simulink model "test"  (R2015a)
settings: Solver=ode45  StartTime=0.0  StopTime=380000  RelTol=1e-3
InitFcn:
  | %% DSPBuilder Start
  | alt_dspbuilder_update_model(bdroot)
  | %% DSPBuilder End
libraries: allblocks_alteradspbuilder2 x2155
(part 1 of 24)
settings Model: Creator=ASUS  LastModifiedBy=ASUS

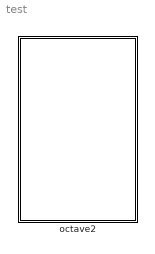
== system test ==
  octave2 : Subsystem

== system test/octave2 ==
  AltBus : allblocks_alteradspbuilder2/AltBus  BusType=Unsigned Integer  bwl=128  bwr=0  saturate=off  floatingPointInput=on  floatingPointOutput=on  logOutputs=off  logFile=C:\Users\ASUS\Desktop\sift_fpga_final\Octave_2\tb_test\test_octave2_AltBus.fixedpointlog
  AltBus1 : allblocks_alteradspbuilder2/AltBus  BusType=Unsigned Integer  bwl=1173  bwr=0  saturate=off  floatingPointInput=on  floatingPointOutput=on  logOutputs=off  logFile=C:\Users\ASUS\Desktop\sift_fpga_final\Octave_2\tb_test\test_octave2_AltBus1.fixedpointlog
  Bus_Concatenation : Subsystem
  Delay : allblocks_alteradspbuilder2/Delay  pipeline=1  pipeline_display=1  ClockPhase=1  use_ena=on  use_sclr=off  allowFloatingPointOverride=on  logOutputs=off  logFile=C:\Users\ASUS\Desktop\sift_fpga_final\Octave_2\tb_test\test_octave2_Delay.fixedpointlog  use_init=off  reset_value=1
  From Workspace : FromWorkspace  VariableName=pixel_in  SampleTime=0
  From Workspace1 : FromWorkspace  VariableName=valid_in  SampleTime=0
  From Workspace2 : FromWorkspace  VariableName=sof_in  SampleTime=0
  From Workspace3 : FromWorkspace  VariableName=eof_in  SampleTime=0
  GradOrien : Subsystem
  Line_buff_11x11 : Subsystem
  Memory Delay : allblocks_alteradspbuilder2/Memory Delay  BusType=Unsigned Integer  bwl=1  bwr=0  pipeline=4495  pipeline_display=4495  ram_type=AUTO  use_ena=off  use_sclr=off  allowFloatingPointOverride=on  logOutputs=off  logFile=C:\Users\ASUS\Desktop\sift_fpga_final\Octave_2\tb_test\test_octave2_Memory+Delay.fixedpointlog
  Memory Delay1 : allblocks_alteradspbuilder2/Memory Delay  BusType=Unsigned Integer  bwl=10  bwr=0  pipeline=6443  pipeline_display=6443  ram_type=AUTO  use_ena=off  use_sclr=off  allowFloatingPointOverride=on  logOutputs=off  logFile=C:\Users\ASUS\Desktop\sift_fpga_final\Octave_2\tb_test\test_octave2_Memory+Delay1.fixedpointlog
  Memory Delay2 : allblocks_alteradspbuilder2/Memory Delay  BusType=Unsigned Integer  bwl=10  bwr=0  pipeline=6443  pipeline_display=6443  ram_type=AUTO  use_ena=off  use_sclr=off  allowFloatingPointOverride=on  logOutputs=off  logFile=C:\Users\ASUS\Desktop\sift_fpga_final\Octave_2\tb_test\test_octave2_Memory+Delay2.fixedpointlog
  Ram : Subsystem
  Ram_location_match : Subsystem
  add_read_desciptor : Subsystem
  calculate_key_point : Subsystem
  compare_descriptor : Subsystem
  counter : Subsystem
  descriptor : Subsystem
  dog_space : Subsystem
  hist_bin : Subsystem
  scale_space : Subsystem
  sink_validIn : allblocks_alteradspbuilder2/Input  iofile=C:\Users\ASUS\Desktop\sift_fpga_final\Octave_2\tb_test\test_octave2_sink%5FvalidIn.salt  BusType=Single Bit  bwl=8  bwr=0  SpecifyClock=off  PORTTYPE=Input  externalType=Inferred  allowFloatingPointOverride=on  logOutputs=off
  sink_validIn1 : allblocks_alteradspbuilder2/Input  iofile=C:\Users\ASUS\Desktop\sift_fpga_final\Octave_2\tb_test\test_octave2_sink%5FvalidIn1.salt  BusType=Single Bit  bwl=8  bwr=0  SpecifyClock=off  PORTTYPE=Input  externalType=Inferred  allowFloatingPointOverride=on  logOutputs=off
  sink_validIn2 : allblocks_alteradspbuilder2/Input  iofile=C:\Users\ASUS\Desktop\sift_fpga_final\Octave_2\tb_test\test_octave2_sink%5FvalidIn2.salt  BusType=Single Bit  bwl=8  bwr=0  SpecifyClock=off  PORTTYPE=Input  externalType=Inferred  allowFloatingPointOverride=on  logOutputs=off
  sink_validIn3 : allblocks_alteradspbuilder2/Input  iofile=C:\Users\ASUS\Desktop\sift_fpga_final\Octave_2\tb_test\test_octave2_sink%5FvalidIn3.salt  BusType=Unsigned Integer  bwl=8  bwr=0  SpecifyClock=off  PORTTYPE=Input  externalType=Inferred  allowFloatingPointOverride=on  logOutputs=off
  wires:
  GradOrien/1(m_xy) -> hist_bin/1(m_xy_In)
  hist_bin/6(hist_bin6_out) -> Bus_Concatenation/6(bin6_in)
  hist_bin/8(hist_bin8_out) -> Bus_Concatenation/8(bin8_in)
  [valid_in] -> scale_space/2(valid_in)
  [valid_in] -> dog_space/5(valid_in)
  scale_space/1(scale4) -> dog_space/1(scale4_in)
  scale_space/3(scale2) -> GradOrien/1(data_in), dog_space/3(scale2_in)
  [valid_in] -> GradOrien/2(clken)
  scale_space/2(scale3) -> dog_space/2(scale3_in)
  scale_space/4(scale1) -> dog_space/4(scale1_in)
  [pixel_in] -> scale_space/1(data_in)
  [valid_in] -> calculate_key_point/4(valid_in)
  dog_space/2(dog2_out) -> calculate_key_point/2(pixel_dog2_in)
  [valid_in] -> hist_bin/3(clken)
  dog_space/1(dog3_out) -> calculate_key_point/1(pixel_dog3_in)
  GradOrien/2(orien) -> hist_bin/2(orien_In)
  dog_space/3(dog1_out) -> calculate_key_point/3(pixel_dog1_in)
  hist_bin/7(hist_bin7_out) -> Bus_Concatenation/7(bin_in)
  Line_buff_11x11/9(Out1010) -> descriptor/9(data_in1010)
  counter/1(col_out) -> [column]
  Line_buff_11x11/1(Out00) -> descriptor/1(data_in00)
  Line_buff_11x11/6(Out510) -> descriptor/6(data_in510)
  Memory Delay1/1 -> descriptor/11(column_in)
  [column] -> Memory Delay1/1
  Line_buff_11x11/3(Out010) -> descriptor/3(data_in010)
  calculate_key_point/1(is_KeyPoint) -> Memory Delay/1
  Line_buff_11x11/7(Out100) -> descriptor/7(data_in100)
  hist_bin/5(hist_bin5_out) -> Bus_Concatenation/5(bin5_in)
  hist_bin/3(hist_bin3_out) -> Bus_Concatenation/3(biin3_in)
  hist_bin/2(hist_bin2_out) -> Bus_Concatenation/2(bin2_in)
  [sof_in] -> counter/3(sof_in)
  counter/2(row_out) -> [row]
  Line_buff_11x11/2(Out05) -> descriptor/2(data_in05)
  hist_bin/1(hist_bin1_out) -> Bus_Concatenation/1(bin1_in)
  [valid_in] -> Line_buff_11x11/2(clken)
  [eof_in] -> counter/2(eof_in)
  hist_bin/4(hist_bin4_out) -> Bus_Concatenation/4(bin4_in)
  [valid_in] -> counter/1(valid_in)
  Line_buff_11x11/4(Out50) -> descriptor/4(data_in50)
  Line_buff_11x11/5(Out55) -> descriptor/5(data_in55)
  Memory Delay/1 -> descriptor/10(isKeyPoint_in)
  Bus_Concatenation/1(hist_bin) -> AltBus/1
  Memory Delay2/1 -> descriptor/12(row_in)
  [row] -> Memory Delay2/1
  Line_buff_11x11/8(Out105) -> descriptor/8(data_in105)
  descriptor/1(descriptor_out) -> AltBus1/1
  From Workspace2/1 -> sink_validIn1/1
  From Workspace/1 -> sink_validIn3/1
  From Workspace3/1 -> sink_validIn/1
  From Workspace1/1 -> sink_validIn2/1
  sink_validIn/1 -> [eof_in]
  sink_validIn1/1 -> [sof_in]
  sink_validIn2/1 -> [valid_in]
  sink_validIn3/1 -> [pixel_in]
  AltBus/1 -> Line_buff_11x11/1(dataIn)
  AltBus1/1 -> Ram/1(descriptor)
  Ram/1(read_out1) -> compare_descriptor/1(descriptor1)
  Ram/2(read_out2) -> compare_descriptor/2(descriptor2)
  add_read_desciptor/1(add_read1) -> Ram/4(add_read1)
  add_read_desciptor/2(add_read2) -> Ram/5(add_read2)
  [valid_in] -> add_read_desciptor/1(valid_in)
  [valid_in] -> compare_descriptor/3(clken)
  compare_descriptor/1(match) -> Ram_location_match/1(match)
  compare_descriptor/2(location) -> Ram_location_match/2(location)
  [valid_in] -> Ram_location_match/3(clken)
  add_read_desciptor/3(rs_ram_location) -> Delay/1
  Delay/1 -> Ram_location_match/4(sclr)
  [valid_in] -> Delay/2

== system test/octave2/Bus_Concatenation ==
  bin1_in : Inport
  bin2_in : Inport  Port=2
  biin3_in : Inport  Port=3
  bin4_in : Inport  Port=4
  bin5_in : Inport  Port=5
  bin6_in : Inport  Port=6
  bin_in : Inport  Port=7
  bin8_in : Inport  Port=8
  Bus Concatenation{,1..3} (4 alike) : allblocks_alteradspbuilder2/Bus Concatenation  isSigned=off  awidth=16  bwidth=16  pipeline_display=0
  Bus Concatenation7 : allblocks_alteradspbuilder2/Bus Concatenation  isSigned=off  awidth=32  bwidth=32  pipeline_display=0
  Bus Concatenation8 : allblocks_alteradspbuilder2/Bus Concatenation  isSigned=off  awidth=32  bwidth=32  pipeline_display=0
  Bus Concatenation9 : allblocks_alteradspbuilder2/Bus Concatenation  isSigned=off  awidth=64  bwidth=64  pipeline_display=0
  hist_bin : Outport
  wires:
  bin1_in/1 -> [bin1]
  bin2_in/1 -> [bin2]
  biin3_in/1 -> [bin3]
  bin4_in/1 -> [bin4]
  bin5_in/1 -> [bin5]
  bin6_in/1 -> [bin6]
  bin_in/1 -> [bin7]
  bin8_in/1 -> [bin8]
  Bus Concatenation/1 -> Bus Concatenation8/2
  [bin6] -> Bus Concatenation1/2
  Bus Concatenation1/1 -> Bus Concatenation8/1
  [bin8] -> Bus Concatenation/2
  [bin5] -> Bus Concatenation1/1
  [bin7] -> Bus Concatenation/1
  Bus Concatenation9/1 -> hist_bin/1
  [bin4] -> Bus Concatenation2/2
  [bin3] -> Bus Concatenation2/1
  [bin2] -> Bus Concatenation3/2
  [bin1] -> Bus Concatenation3/1
  Bus Concatenation3/1 -> Bus Concatenation7/1
  Bus Concatenation2/1 -> Bus Concatenation7/2
  Bus Concatenation7/1 -> Bus Concatenation9/1
  Bus Concatenation8/1 -> Bus Concatenation9/2

== system test/octave2/GradOrien ==
  data_in : Inport
  clken : Inport  Port=2
  lineBuff_3x3 : Subsystem
  sub_GradOrian : Subsystem
  m_xy : Outport
  orien : Outport  Port=2
  wires:
  sub_GradOrian/1(orien) -> orien/1
  clken/1 -> sub_GradOrian/5(clken), lineBuff_3x3/2(clken)
  data_in/1 -> lineBuff_3x3/1(dataIn)
  sub_GradOrian/2(m_xy) -> m_xy/1
  lineBuff_3x3/1(Out01) -> sub_GradOrian/1(L_y_add_1)
  lineBuff_3x3/4(Out21) -> sub_GradOrian/4(L_y_sub_1)
  lineBuff_3x3/3(Out12) -> sub_GradOrian/3(L_x_sub_1)
  lineBuff_3x3/2(Out10) -> sub_GradOrian/2(L_x_add_1)

== system test/octave2/Line_buff_11x11 ==
  dataIn : Inport
  clken : Inport  Port=2
  Memory Delay1 : allblocks_alteradspbuilder2/Memory Delay  BusType=Unsigned Integer  bwl=128  bwr=0  pipeline=1  pipeline_display=1  ram_type=AUTO  use_ena=on  use_sclr=off  allowFloatingPointOverride=on  logOutputs=off  logFile=C:\Users\ASUS\Desktop\sift_fpga_final\Octave_2\tb_test\test_octave2_Line%5Fbuff%5F11x11_Memory+Delay1.fixedpointlog
  Memory Delay11 : allblocks_alteradspbuilder2/Memory Delay  BusType=Unsigned Integer  bwl=128  bwr=0  pipeline=630  pipeline_display=630  ram_type=AUTO  use_ena=on  use_sclr=off  allowFloatingPointOverride=on  logOutputs=off  logFile=C:\Users\ASUS\Desktop\sift_fpga_final\Octave_2\tb_test\test_octave2_Line%5Fbuff%5F11x11_Memory+Delay11.fixedpointlog
  Memory Delay12 : allblocks_alteradspbuilder2/Memory Delay  BusType=Unsigned Integer  bwl=128  bwr=0  pipeline=5  pipeline_display=5  ram_type=AUTO  use_ena=on  use_sclr=off  allowFloatingPointOverride=on  logOutputs=off  logFile=C:\Users\ASUS\Desktop\sift_fpga_final\Octave_2\tb_test\test_octave2_Line%5Fbuff%5F11x11_Memory+Delay12.fixedpointlog
  Memory Delay13 : allblocks_alteradspbuilder2/Memory Delay  BusType=Unsigned Integer  bwl=128  bwr=0  pipeline=5  pipeline_display=5  ram_type=AUTO  use_ena=on  use_sclr=off  allowFloatingPointOverride=on  logOutputs=off  logFile=C:\Users\ASUS\Desktop\sift_fpga_final\Octave_2\tb_test\test_octave2_Line%5Fbuff%5F11x11_Memory+Delay13.fixedpointlog
  Memory Delay15 : allblocks_alteradspbuilder2/Memory Delay  BusType=Unsigned Integer  bwl=128  bwr=0  pipeline=630  pipeline_display=630  ram_type=AUTO  use_ena=on  use_sclr=off  allowFloatingPointOverride=on  logOutputs=off  logFile=C:\Users\ASUS\Desktop\sift_fpga_final\Octave_2\tb_test\test_octave2_Line%5Fbuff%5F11x11_Memory+Delay15.fixedpointlog
  Memory Delay16 : allblocks_alteradspbuilder2/Memory Delay  BusType=Unsigned Integer  bwl=128  bwr=0  pipeline=5  pipeline_display=5  ram_type=AUTO  use_ena=on  use_sclr=off  allowFloatingPointOverride=on  logOutputs=off  logFile=C:\Users\ASUS\Desktop\sift_fpga_final\Octave_2\tb_test\test_octave2_Line%5Fbuff%5F11x11_Memory+Delay16.fixedpointlog
  Memory Delay17 : allblocks_alteradspbuilder2/Memory Delay  BusType=Unsigned Integer  bwl=128  bwr=0  pipeline=5  pipeline_display=5  ram_type=AUTO  use_ena=on  use_sclr=off  allowFloatingPointOverride=on  logOutputs=off  logFile=C:\Users\ASUS\Desktop\sift_fpga_final\Octave_2\tb_test\test_octave2_Line%5Fbuff%5F11x11_Memory+Delay17.fixedpointlog
  Memory Delay18 : allblocks_alteradspbuilder2/Memory Delay  BusType=Unsigned Integer  bwl=128  bwr=0  pipeline=640*4  pipeline_display=2560  ram_type=AUTO  use_ena=on  use_sclr=off  allowFloatingPointOverride=on  logOutputs=off  logFile=C:\Users\ASUS\Desktop\sift_fpga_final\Octave_2\tb_test\test_octave2_Line%5Fbuff%5F11x11_Memory+Delay18.fixedpointlog
  Memory Delay5 : allblocks_alteradspbuilder2/Memory Delay  BusType=Unsigned Integer  bwl=128  bwr=0  pipeline=5  pipeline_display=5  ram_type=AUTO  use_ena=on  use_sclr=off  allowFloatingPointOverride=on  logOutputs=off  logFile=C:\Users\ASUS\Desktop\sift_fpga_final\Octave_2\tb_test\test_octave2_Line%5Fbuff%5F11x11_Memory+Delay5.fixedpointlog
  Memory Delay6 : allblocks_alteradspbuilder2/Memory Delay  BusType=Unsigned Integer  bwl=128  bwr=0  pipeline=5  pipeline_display=5  ram_type=AUTO  use_ena=on  use_sclr=off  allowFloatingPointOverride=on  logOutputs=off  logFile=C:\Users\ASUS\Desktop\sift_fpga_final\Octave_2\tb_test\test_octave2_Line%5Fbuff%5F11x11_Memory+Delay6.fixedpointlog
  Memory Delay7 : allblocks_alteradspbuilder2/Memory Delay  BusType=Unsigned Integer  bwl=128  bwr=0  pipeline=640*4  pipeline_display=2560  ram_type=AUTO  use_ena=on  use_sclr=off  allowFloatingPointOverride=on  logOutputs=off  logFile=C:\Users\ASUS\Desktop\sift_fpga_final\Octave_2\tb_test\test_octave2_Line%5Fbuff%5F11x11_Memory+Delay7.fixedpointlog
  Out00 : Outport
  Out05 : Outport  Port=2
  Out010 : Outport  Port=3
  Out50 : Outport  Port=4
  Out55 : Outport  Port=5
  Out510 : Outport  Port=6
  Out100 : Outport  Port=7
  Out105 : Outport  Port=8
  Out1010 : Outport  Port=9
  wires:
  [clken] -> Memory Delay11/2
  [clken] -> Memory Delay17/2
  [clken] -> Memory Delay6/2
  Memory Delay6/1 -> [data_010], Memory Delay7/1
  [clken] -> Memory Delay18/2
  Memory Delay18/1 -> Memory Delay15/1
  Memory Delay13/1 -> Memory Delay18/1, [data_510]
  [clken] -> Memory Delay15/2
  [clken] -> Memory Delay16/2
  Memory Delay17/1 -> [data_1010]
  Memory Delay16/1 -> Memory Delay17/1, [data_105]
  Memory Delay15/1 -> Memory Delay16/1, [data_100]
  [clken] -> Memory Delay7/2
  [clken] -> Memory Delay12/2
  Memory Delay11/1 -> Memory Delay12/1, [data_50]
  Memory Delay12/1 -> Memory Delay13/1, [data_55]
  Memory Delay7/1 -> Memory Delay11/1
  [clken] -> Memory Delay13/2
  [data_55] -> Out55/1
  [data_010] -> Out010/1
  [data_05] -> Out05/1
  clken/1 -> [clken]
  [data_00] -> Out00/1
  [data_50] -> Out50/1
  [data_100] -> Out100/1
  [data_510] -> Out510/1
  [data_1010] -> Out1010/1
  dataIn/1 -> [data_in]
  [data_105] -> Out105/1
  [clken] -> Memory Delay5/2
  Memory Delay1/1 -> Memory Delay5/1, [data_00]
  [clken] -> Memory Delay1/2
  [data_in] -> Memory Delay1/1
  Memory Delay5/1 -> Memory Delay6/1, [data_05]

== system test/octave2/Ram ==
  descriptor : Inport
  select : Inport  Port=2
  eof : Inport  Port=3
  add_read1 : Inport  Port=4
  add_read2 : Inport  Port=5
  Demultiplexer : allblocks_alteradspbuilder2/Demultiplexer  numOutputs=2  pipeline_display=1  use_ena=off  use_sclr=off  allowFloatingPointOverride=on  logOutputs=off  logFile=C:\Users\ASUS\Desktop\sift_fpga_final\Octave_2\tb_test\test_octave2_Ram_Demultiplexer%3A%3Aq.fixedpointlog,C:\Users\ASUS\Desktop\sift_fpga_final\Octave_2\tb_test\test_octave2_Ram_Demultiplexer%3A%3Aq.fixedpointlog,
  Dual-Port RAM : allblocks_alteradspbuilder2/Dual-Port RAM  numwords=1000  BusType=Signed Integer  bwl=1172  bwr=0  memory_type=AUTO  ram_type=DualRAM  dont_care=on  initialization=Blank  init_file=input.hex  init_array=[0:1:15]  register_outputs=on  use_ena=off  ClockPhase=1  allowFloatingPointOverride=on  logOutputs=off  logFile=C:\Users\ASUS\Desktop\sift_fpga_final\Octave_2\tb_test\test_octave2_Ram_Dual-Port+RAM.fixedpointlog  pipeline_display=2
  Dual-Port RAM1 : allblocks_alteradspbuilder2/Dual-Port RAM  numwords=1000  BusType=Signed Integer  bwl=1172  bwr=0  memory_type=AUTO  ram_type=DualRAM  dont_care=on  initialization=Blank  init_file=input.hex  init_array=[0:1:15]  register_outputs=on  use_ena=off  ClockPhase=1  allowFloatingPointOverride=on  logOutputs=off  logFile=C:\Users\ASUS\Desktop\sift_fpga_final\Octave_2\tb_test\test_octave2_Ram_Dual-Port+RAM1.fixedpointlog  pipeline_display=2
  Subsystem : Subsystem
  Subsystem1 : Subsystem
  read_out1 : Outport
  read_out2 : Outport  Port=2
  wires:
  Demultiplexer/1 -> Subsystem/1(descriptor)
  [descriptor] -> Demultiplexer/1
  Subsystem/2(add_write) -> Dual-Port RAM/3
  Subsystem/1(data) -> Dual-Port RAM/1
  Subsystem/3(ena_write) -> Dual-Port RAM/4
  [eof] -> Subsystem1/2(eof)
  [add_read1] -> Dual-Port RAM/2
  Dual-Port RAM/1 -> read_out1/1
  Dual-Port RAM1/1 -> read_out2/1
  [add_read2] -> Dual-Port RAM1/2
  [eof] -> Subsystem/2(eof)
  Demultiplexer/2 -> Subsystem1/1(descriptor)
  Subsystem1/1(data) -> Dual-Port RAM1/1
  Subsystem1/2(add_write) -> Dual-Port RAM1/3
  Subsystem1/3(ena_write) -> Dual-Port RAM1/4
  eof/1 -> [eof]
  select/1 -> [select]
  [select] -> Demultiplexer/2
  descriptor/1 -> [descriptor]
  add_read1/1 -> [add_read1]
  add_read2/1 -> [add_read2]

== system test/octave2/Ram_location_match ==
  match : Inport
  location : Inport  Port=2
  clken : Inport  Port=3
  sclr : Inport  Port=4
  Counter : allblocks_alteradspbuilder2/Counter  BusType=Unsigned Integer  bwl=10  bwr=0  use_modulo=on  modulo=1000  SpecifyClock=off  direction=Increment  use_sload=off  use_sset=off  svalue=1  use_clk_ena=off  use_ena=on  use_sclr=on  pipeline_display=1
  Dual-Port RAM : allblocks_alteradspbuilder2/Dual-Port RAM  numwords=1000  BusType=Signed Integer  bwl=20  bwr=0  memory_type=AUTO  ram_type=DualRAM  dont_care=on  initialization=Blank  init_file=input.hex  init_array=[0:1:15]  register_outputs=on  use_ena=off  ClockPhase=1  allowFloatingPointOverride=on  logOutputs=off  logFile=C:\Users\ASUS\Desktop\sift_fpga_final\Octave_2\tb_test\test_octave2_Ram%5Flocation%5Fmatch_Dual-Port+RAM.fixedpointlog  pipeline_display=2
  Logical Bit Operator : allblocks_alteradspbuilder2/Logical Bit Operator  LogicalOperator=AND  user_inputs=2  pipeline_display=0
  Logical Bit Operator1 : allblocks_alteradspbuilder2/Logical Bit Operator  LogicalOperator=AND  user_inputs=2  pipeline_display=0
  Logical Bit Operator2 : allblocks_alteradspbuilder2/Logical Bit Operator  LogicalOperator=AND  user_inputs=2  pipeline_display=0
  wires:
  match/1 -> [match]
  location/1 -> [location]
  clken/1 -> [clken]
  Logical Bit Operator/1 -> Counter/1
  Counter/1 -> [add_write]
  [match] -> Logical Bit Operator/2
  [clken] -> Logical Bit Operator/1
  [location] -> Dual-Port RAM/1
  [add_write] -> Dual-Port RAM/3
  Logical Bit Operator1/1 -> Dual-Port RAM/4
  [match] -> Logical Bit Operator1/2
  [clken] -> Logical Bit Operator1/1
  sclr/1 -> [sclr]
  [sclr] -> Logical Bit Operator2/2
  [clken] -> Logical Bit Operator2/1
  Logical Bit Operator2/1 -> Counter/2

== system test/octave2/add_read_desciptor ==
  valid_in : Inport
  option_ena : Inport  Port=2
  Comparator : allblocks_alteradspbuilder2/Comparator  direction=a == b  pipeline_display=0  allowFloatingPointOverride=on  logOutputs=off  logFile=C:\Users\ASUS\Desktop\sift_fpga_final\Octave_2\tb_test\test_octave2_add%5Fread%5Fdesciptor_Comparator.fixedpointlog
  Comparator1 : allblocks_alteradspbuilder2/Comparator  direction=a == b  pipeline_display=0  allowFloatingPointOverride=on  logOutputs=off  logFile=C:\Users\ASUS\Desktop\sift_fpga_final\Octave_2\tb_test\test_octave2_add%5Fread%5Fdesciptor_Comparator1.fixedpointlog
  Constant : allblocks_alteradspbuilder2/Constant  mask_cst=999  BusType=Unsigned Integer  bwl=10  bwr=0  roundMode=Truncate  satMode=Wrap  SpecifyClock=off  allowFloatingPointOverride=on  logOutputs=off  logFile=C:\Users\ASUS\Desktop\sift_fpga_final\Octave_2\tb_test\test_octave2_add%5Fread%5Fdesciptor_Constant.fixedpointlog
  Constant1 : allblocks_alteradspbuilder2/Constant  mask_cst=999  BusType=Unsigned Integer  bwl=10  bwr=0  roundMode=Truncate  satMode=Wrap  SpecifyClock=off  allowFloatingPointOverride=on  logOutputs=off  logFile=C:\Users\ASUS\Desktop\sift_fpga_final\Octave_2\tb_test\test_octave2_add%5Fread%5Fdesciptor_Constant1.fixedpointlog
  Counter : allblocks_alteradspbuilder2/Counter  BusType=Unsigned Integer  bwl=10  bwr=0  use_modulo=on  modulo=1000  SpecifyClock=off  direction=Increment  use_sload=off  use_sset=off  svalue=1  use_clk_ena=off  use_ena=on  use_sclr=off  pipeline_display=1
  Counter1 : allblocks_alteradspbuilder2/Counter  BusType=Unsigned Integer  bwl=10  bwr=0  use_modulo=on  modulo=1000  SpecifyClock=off  direction=Increment  use_sload=off  use_sset=off  svalue=0  use_clk_ena=off  use_ena=on  use_sclr=off  pipeline_display=1
  Logical Bit Operator : allblocks_alteradspbuilder2/Logical Bit Operator  LogicalOperator=AND  user_inputs=2  pipeline_display=0
  Logical Bit Operator1 : allblocks_alteradspbuilder2/Logical Bit Operator  LogicalOperator=AND  user_inputs=2  pipeline_display=0
  add_read1 : Outport
  add_read2 : Outport  Port=2
  rs_ram_location : Outport  Port=3
  wires:
  Logical Bit Operator/1 -> Counter1/1
  [counter_col] -> Comparator/1
  option_ena/1 -> [ena]
  Constant/1 -> Comparator/2
  Comparator/1 -> Logical Bit Operator/2
  valid_in/1 -> [valid_in]
  Counter1/1 -> [add_read2]
  Counter/1 -> [add_read1]
  Logical Bit Operator1/1 -> Logical Bit Operator/1, Counter/1
  [add_read2] -> add_read2/1
  [add_read1] -> add_read1/1
  [ena] -> Logical Bit Operator1/1
  [valid_in] -> Logical Bit Operator1/2
  [add_read2] -> Comparator1/1
  Constant1/1 -> Comparator1/2
  Comparator1/1 -> [reset_add_ram_location_match]
  [reset_add_ram_location_match] -> rs_ram_location/1

== system test/octave2/calculate_key_point ==
  pixel_dog3_in : Inport
  pixel_dog2_in : Inport  Port=2
  pixel_dog1_in : Inport  Port=3
  valid_in : Inport  Port=4
  find_KeyPoint : Subsystem
  line_buff_3x3 : Subsystem
  line_buff_3x3(1) : Subsystem
  line_buff_3x3(2) : Subsystem
  is_KeyPoint : Outport
  wires:
  line_buff_3x3/3(Out02) -> find_KeyPoint/3(dataIn_12)
  line_buff_3x3/6(Out12) -> find_KeyPoint/6(dataIn_15)
  line_buff_3x3/4(Out10) -> find_KeyPoint/4(dataIn_13)
  line_buff_3x3/5(Out11) -> find_KeyPoint/5(dataIn_14)
  line_buff_3x3(1)/2(Out01) -> find_KeyPoint/11(dataIn_21)
  line_buff_3x3(1)/3(Out02) -> find_KeyPoint/12(dataIn_22)
  line_buff_3x3(1)/4(Out10) -> find_KeyPoint/13(dataIn_23)
  line_buff_3x3/2(Out01) -> find_KeyPoint/2(dataIn_11)
  line_buff_3x3(2)/8(Out21) -> find_KeyPoint/26(dataIn_37)
  line_buff_3x3/8(Out21) -> find_KeyPoint/8(dataIn_17)
  line_buff_3x3/1(Out00) -> find_KeyPoint/1(dataIn_10)
  line_buff_3x3/7(Out20) -> find_KeyPoint/7(dataIn_16)
  line_buff_3x3/9(Out22) -> find_KeyPoint/9(dataIn_18)
  line_buff_3x3(1)/1(Out00) -> find_KeyPoint/10(dataIn_20)
  line_buff_3x3(2)/7(Out20) -> find_KeyPoint/25(dataIn_36)
  [pixel_dog2_in] -> line_buff_3x3(1)/1(dataIn)
  [pixel_dog1_in] -> line_buff_3x3/1(dataIn)
  [valid_in] -> line_buff_3x3(2)/2(clken)
  valid_in/1 -> [valid_in]
  [valid_in] -> line_buff_3x3(1)/2(clken)
  pixel_dog2_in/1 -> [pixel_dog2_in]
  pixel_dog1_in/1 -> [pixel_dog1_in]
  pixel_dog3_in/1 -> [pixel_dog3_in]
  [valid_in] -> line_buff_3x3/2(clken)
  [pixel_dog3_in] -> line_buff_3x3(2)/1(dataIn)
  line_buff_3x3(2)/2(Out01) -> find_KeyPoint/20(dataIn_31)
  line_buff_3x3(2)/3(Out02) -> find_KeyPoint/21(dataIn_32)
  line_buff_3x3(2)/4(Out10) -> find_KeyPoint/22(dataIn_33)
  line_buff_3x3(2)/5(Out11) -> find_KeyPoint/23(dataIn_34)
  line_buff_3x3(2)/1(Out00) -> find_KeyPoint/19(dataIn_30)
  line_buff_3x3(1)/5(Out11) -> find_KeyPoint/14(dataIn_24)
  line_buff_3x3(1)/6(Out12) -> find_KeyPoint/15(dataIn_25)
  line_buff_3x3(1)/7(Out20) -> find_KeyPoint/16(dataIn_26)
  line_buff_3x3(1)/8(Out21) -> find_KeyPoint/17(dataIn_27)
  line_buff_3x3(2)/6(Out12) -> find_KeyPoint/24(dataIn_35)
  line_buff_3x3(2)/9(Out22) -> find_KeyPoint/27(dataIn_38)
  line_buff_3x3(1)/9(Out22) -> find_KeyPoint/18(dataIn_28)
  find_KeyPoint/1(is_KeyPoint) -> is_KeyPoint/1

== system test/octave2/compare_descriptor ==
  descriptor1 : Inport
  descriptor2 : Inport  Port=2
  clken : Inport  Port=3
  threshold : Inport  Port=4
  AltBus1 : allblocks_alteradspbuilder2/AltBus  BusType=Unsigned Integer  bwl=20  bwr=0  saturate=off  floatingPointInput=on  floatingPointOutput=on  logOutputs=off  logFile=C:\Users\ASUS\Desktop\sift_fpga_final\Octave_2\tb_test\test_octave2_compare%5Fdescriptor_AltBus1.fixedpointlog
  BusSplitter : Subsystem
  BusSplitter1 : Subsystem
  Logical Bus Operator : allblocks_alteradspbuilder2/Logical Bus Operator  BusType=Unsigned Integer  bwl=1173  bwr=0  LogicalOp_text=AND  mask_value_num=128*9  shift_amount=3  force_sign_ext=on  pipeline_display=0
  Parallel Adder Subtractor : allblocks_alteradspbuilder2/Parallel Adder Subtractor  number_of_inputs=9  direction=+  use_pipeline=on  pipeline_display=4  phase_selection=1  use_ena=on  use_aclr=off  allowFloatingPointOverride=on  logOutputs=off  logFile=C:\Users\ASUS\Desktop\sift_fpga_final\Octave_2\tb_test\test_octave2_compare%5Fdescriptor_Parallel+Adder+Subtractor.fixedpointlog
  compare : Subsystem
  get_distance : Subsystem
  get_distance1 : Subsystem
  get_distance2 : Subsystem
  get_distance3 : Subsystem
  get_distance4 : Subsystem
  get_distance5 : Subsystem
  get_distance6 : Subsystem
  get_distance7 : Subsystem
  get_distance8 : Subsystem
  match : Outport
  location : Outport  Port=2
  wires:
  descriptor1/1 -> [descriptor1]
  descriptor2/1 -> [descriptor2]
  [descriptor1] -> BusSplitter/1(descriptor_in)
  [descriptor2] -> BusSplitter1/1(descriptor_in)
  BusSplitter/1(hist1) -> [hist11]
  BusSplitter/2(hist2) -> [hist12]
  BusSplitter/3(hist3) -> [hist13]
  BusSplitter/4(hist4) -> [hist14]
  BusSplitter/5(hist5) -> [hist15]
  BusSplitter/6(hist6) -> [hist16]
  BusSplitter/7(hist7) -> [hist17]
  BusSplitter/8(hist8) -> [hist18]
  BusSplitter/9(hist9) -> [hist19]
  BusSplitter1/1(hist1) -> [hist21]
  BusSplitter1/2(hist2) -> [hist22]
  BusSplitter1/3(hist3) -> [hist23]
  BusSplitter1/4(hist4) -> [hist24]
  BusSplitter1/5(hist5) -> [hist25]
  BusSplitter1/6(hist6) -> [hist26]
  BusSplitter1/7(hist7) -> [hist27]
  BusSplitter1/8(hist8) -> [hist28]
  BusSplitter1/9(hist9) -> [hist29]
  clken/1 -> [clken]
  [clken] -> get_distance/3(clken)
  [hist21] -> get_distance/2(hist_in2)
  [hist11] -> get_distance/1(hist_in1)
  get_distance/1(distance_out) -> [distance1]
  [clken] -> get_distance1/3(clken)
  [hist22] -> get_distance1/2(hist_in2)
  [hist12] -> get_distance1/1(hist_in1)
  get_distance1/1(distance_out) -> [distance2]
  [clken] -> get_distance2/3(clken)
  [hist23] -> get_distance2/2(hist_in2)
  [hist13] -> get_distance2/1(hist_in1)
  get_distance2/1(distance_out) -> [distance3]
  [clken] -> get_distance3/3(clken)
  [hist24] -> get_distance3/2(hist_in2)
  [hist14] -> get_distance3/1(hist_in1)
  get_distance3/1(distance_out) -> [distance4]
  [clken] -> get_distance4/3(clken)
  [hist25] -> get_distance4/2(hist_in2)
  [hist15] -> get_distance4/1(hist_in1)
  get_distance4/1(distance_out) -> [distance5]
  [clken] -> get_distance5/3(clken)
  [hist26] -> get_distance5/2(hist_in2)
  [hist16] -> get_distance5/1(hist_in1)
  get_distance5/1(distance_out) -> [distance6]
  [clken] -> get_distance6/3(clken)
  [hist27] -> get_distance6/2(hist_in2)
  [hist17] -> get_distance6/1(hist_in1)
  get_distance6/1(distance_out) -> [distance7]
  [clken] -> get_distance7/3(clken)
  [hist28] -> get_distance7/2(hist_in2)
  [hist18] -> get_distance7/1(hist_in1)
  get_distance7/1(distance_out) -> [distance8]
  [clken] -> get_distance8/3(clken)
  [hist29] -> get_distance8/2(hist_in2)
  [hist19] -> get_distance8/1(hist_in1)
  get_distance8/1(distance_out) -> [distance9]
  [distance1] -> Parallel Adder Subtractor/1
  [distance2] -> Parallel Adder Subtractor/2
  [distance3] -> Parallel Adder Subtractor/3
  [distance4] -> Parallel Adder Subtractor/4
  [distance5] -> Parallel Adder Subtractor/5
  [distance6] -> Parallel Adder Subtractor/6
  [distance7] -> Parallel Adder Subtractor/7
  [distance8] -> Parallel Adder Subtractor/8
  [distance9] -> Parallel Adder Subtractor/9
  [clken] -> Parallel Adder Subtractor/10
  Parallel Adder Subtractor/1 -> [distance]
  threshold/1 -> [threshold]
  [distance] -> compare/2(distance)
  [threshold] -> compare/1(threshold)
  compare/1(match) -> [match]
  [descriptor2] -> Logical Bus Operator/1
  Logical Bus Operator/1 -> AltBus1/1
  AltBus1/1 -> [location]
  [location] -> location/1
  [match] -> match/1

== system test/octave2/counter ==
  valid_in : Inport
  eof_in : Inport  Port=2
  sof_in : Inport  Port=3
  Comparator : allblocks_alteradspbuilder2/Comparator  direction=a == b  pipeline_display=0  allowFloatingPointOverride=on  logOutputs=off  logFile=C:\Users\ASUS\Desktop\sift_fpga_final\Octave_2\tb_test\test_octave2_counter_Comparator.fixedpointlog
  Constant : allblocks_alteradspbuilder2/Constant  mask_cst=639  BusType=Unsigned Integer  bwl=10  bwr=0  roundMode=Truncate  satMode=Wrap  SpecifyClock=off  allowFloatingPointOverride=on  logOutputs=off  logFile=C:\Users\ASUS\Desktop\sift_fpga_final\Octave_2\tb_test\test_octave2_counter_Constant.fixedpointlog
  Counter : allblocks_alteradspbuilder2/Counter  BusType=Unsigned Integer  bwl=10  bwr=0  use_modulo=on  modulo=640  SpecifyClock=off  direction=Increment  use_sload=off  use_sset=on  svalue=1  use_clk_ena=off  use_ena=on  use_sclr=on  pipeline_display=1
  Counter1 : allblocks_alteradspbuilder2/Counter  BusType=Unsigned Integer  bwl=10  bwr=0  use_modulo=on  modulo=480  SpecifyClock=off  direction=Increment  use_sload=off  use_sset=on  svalue=0  use_clk_ena=off  use_ena=on  use_sclr=on  pipeline_display=1
  Logical Bit Operator : allblocks_alteradspbuilder2/Logical Bit Operator  LogicalOperator=AND  user_inputs=2  pipeline_display=0
  col_out : Outport
  row_out : Outport  Port=2
  wires:
  [sof_in] -> Counter1/1, Counter/1
  [eof_in] -> Counter1/3
  Logical Bit Operator/1 -> Counter1/2
  [counter_col] -> Comparator/1
  eof_in/1 -> [eof_in]
  Constant/1 -> Comparator/2
  Comparator/1 -> Logical Bit Operator/2
  valid_in/1 -> [valid_in]
  Counter1/1 -> [counter_row]
  Counter/1 -> [counter_col]
  [valid_in] -> Counter/2, Logical Bit Operator/1
  [counter_row] -> row_out/1
  sof_in/1 -> [sof_in]
  [counter_col] -> col_out/1
  [eof_in] -> Counter/3

== system test/octave2/descriptor ==
  data_in00 : Inport
  data_in05 : Inport  Port=2
  data_in010 : Inport  Port=3
  data_in50 : Inport  Port=4
  data_in55 : Inport  Port=5
  data_in510 : Inport  Port=6
  data_in100 : Inport  Port=7
  data_in105 : Inport  Port=8
  data_in1010 : Inport  Port=9
  isKeyPoint_in : Inport  Port=10
  column_in : Inport  Port=11
  row_in : Inport  Port=12
  AltBus : allblocks_alteradspbuilder2/AltBus  BusType=Unsigned Integer  bwl=128*9  bwr=0  saturate=off  floatingPointInput=on  floatingPointOutput=on  logOutputs=off  logFile=C:\Users\ASUS\Desktop\sift_fpga_final\Octave_2\tb_test\test_octave2_descriptor_AltBus.fixedpointlog
  AltBus1 : allblocks_alteradspbuilder2/AltBus  BusType=Single Bit  bwl=1  bwr=0  saturate=off  floatingPointInput=on  floatingPointOutput=on  logOutputs=off  logFile=C:\Users\ASUS\Desktop\sift_fpga_final\Octave_2\tb_test\test_octave2_descriptor_AltBus1.fixedpointlog
  AltBus2 : allblocks_alteradspbuilder2/AltBus  BusType=Single Bit  bwl=1  bwr=0  saturate=off  floatingPointInput=on  floatingPointOutput=on  logOutputs=off  logFile=C:\Users\ASUS\Desktop\sift_fpga_final\Octave_2\tb_test\test_octave2_descriptor_AltBus2.fixedpointlog
  AltBus3 : allblocks_alteradspbuilder2/AltBus  BusType=Unsigned Integer  bwl=10  bwr=0  saturate=off  floatingPointInput=on  floatingPointOutput=on  logOutputs=off  logFile=C:\Users\ASUS\Desktop\sift_fpga_final\Octave_2\tb_test\test_octave2_descriptor_AltBus3.fixedpointlog
  AltBus4 : allblocks_alteradspbuilder2/AltBus  BusType=Unsigned Integer  bwl=10  bwr=0  saturate=off  floatingPointInput=on  floatingPointOutput=on  logOutputs=off  logFile=C:\Users\ASUS\Desktop\sift_fpga_final\Octave_2\tb_test\test_octave2_descriptor_AltBus4.fixedpointlog
  Bus Concatenation : allblocks_alteradspbuilder2/Bus Concatenation  isSigned=off  awidth=1  bwidth=128*9  pipeline_display=0
  Bus Concatenation1 : allblocks_alteradspbuilder2/Bus Concatenation  isSigned=off  awidth=10  bwidth=10  pipeline_display=0
  Bus Concatenation2 : allblocks_alteradspbuilder2/Bus Concatenation  isSigned=off  awidth=1153  bwidth=20  pipeline_display=0
  BusSplitter : Subsystem
  Constant : allblocks_alteradspbuilder2/Constant  mask_cst=0  BusType=Unsigned Integer  bwl=1152  bwr=0  roundMode=Truncate  satMode=Wrap  SpecifyClock=off  allowFloatingPointOverride=on  logOutputs=off  logFile=C:\Users\ASUS\Desktop\sift_fpga_final\Octave_2\tb_test\test_octave2_descriptor_Constant.fixedpointlog
  Multiplexer : allblocks_alteradspbuilder2/Multiplexer  numInputs=2  pipeline=0  oneHot=off  pipeline_display=0  use_ena=off  use_aclr=off  allowFloatingPointOverride=on  logOutputs=off  logFile=C:\Users\ASUS\Desktop\sift_fpga_final\Octave_2\tb_test\test_octave2_descriptor_Multiplexer.fixedpointlog
  Multiplexer3 : allblocks_alteradspbuilder2/Multiplexer  numInputs=8  pipeline=0  oneHot=off  pipeline_display=0  use_ena=off  use_aclr=off  allowFloatingPointOverride=on  logOutputs=off  logFile=C:\Users\ASUS\Desktop\sift_fpga_final\Octave_2\tb_test\test_octave2_descriptor_Multiplexer3.fixedpointlog
  To Workspace : ToWorkspace  VariableName=descriptor  SaveFormat=Timeseries  SampleTime=-1
  To Workspace1 : ToWorkspace  VariableName=column  SaveFormat=Timeseries  SampleTime=-1
  To Workspace2 : ToWorkspace  VariableName=row  SaveFormat=Timeseries  SampleTime=-1
  To Workspace3 : ToWorkspace  VariableName=isKeyPoint  SaveFormat=Timeseries  SampleTime=-1
  descriptor : Subsystem
  findMax : Subsystem
  descriptor_out : Outport
  wires:
  [hist_105] -> descriptor/8(data_in8)
  [hist_100] -> descriptor/7(data_in7)
  [hist_510] -> descriptor/6(data_in6)
  [hist_55] -> descriptor/5(data_in5)
  Multiplexer3/1 -> AltBus/1
  [hist_1010] -> descriptor/9(data_in9)
  descriptor/1(descriptor1) -> Multiplexer3/2
  [hist_05] -> descriptor/2(data_in2)
  [hist_010] -> descriptor/3(data_in3)
  [hist_50] -> descriptor/4(data_in4)
  descriptor/5(descriptor5) -> Multiplexer3/6
  descriptor/4(descriptor4) -> Multiplexer3/5
  [hist_00] -> descriptor/1(data_in1)
  descriptor/7(descriptor7) -> Multiplexer3/8
  descriptor/8(descriptor8) -> Multiplexer3/9
  descriptor/2(descriptor2) -> Multiplexer3/3
  descriptor/3(descriptor3) -> Multiplexer3/4
  descriptor/6(descriptor6) -> Multiplexer3/7
  BusSplitter/3(bin3) -> findMax/3(bin3)
  data_in00/1 -> [hist_00]
  data_in50/1 -> [hist_50]
  BusSplitter/1(bin1) -> findMax/1(bin1)
  data_in100/1 -> [hist_100]
  data_in010/1 -> [hist_010]
  data_in105/1 -> [hist_105]
  [hist_55] -> BusSplitter/1(data_in)
  data_in510/1 -> [hist_510]
  column_in/1 -> [column]
  data_in1010/1 -> [hist_1010]
  BusSplitter/8(bin8) -> findMax/8(bin8)
  data_in55/1 -> [hist_55]
  isKeyPoint_in/1 -> [isKeyPoint]
  row_in/1 -> [row]
  BusSplitter/4(bin4) -> findMax/4(bin4)
  BusSplitter/2(bin2) -> findMax/2(bin2)
  data_in05/1 -> [hist_05]
  BusSplitter/5(bin5) -> findMax/5(bin5)
  BusSplitter/7(bin7) -> findMax/7(bin7)
  BusSplitter/6(bin6) -> findMax/6(bin6)
  AltBus/1 -> [descriptor]
  [isKeyPoint] -> AltBus1/1
  [column] -> AltBus3/1
  [row] -> AltBus4/1
  [descriptor] -> Bus Concatenation/2
  Bus Concatenation/1 -> Bus Concatenation2/1
  Bus Concatenation1/1 -> Bus Concatenation2/2
  Bus Concatenation2/1 -> descriptor_out/1
  [isKeyPoint] -> AltBus2/1
  AltBus2/1 -> Multiplexer/1
  [descriptor] -> Multiplexer/3
  Constant/1 -> Multiplexer/2
  Multiplexer/1 -> To Workspace/1
  AltBus3/1 -> To Workspace1/1, Bus Concatenation1/1
  AltBus4/1 -> To Workspace2/1, Bus Concatenation1/2
  AltBus1/1 -> To Workspace3/1, Bus Concatenation/1
  findMax/1(bin_max) -> Multiplexer3/1

== system test/octave2/dog_space ==
  scale4_in : Inport
  scale3_in : Inport  Port=2
  scale2_in : Inport  Port=3
  scale1_in : Inport  Port=4
  valid_in : Inport  Port=5
  Parallel Adder Subtractor : allblocks_alteradspbuilder2/Parallel Adder Subtractor  number_of_inputs=2  direction=+-  use_pipeline=on  pipeline_display=1  phase_selection=1  use_ena=on  use_aclr=off  allowFloatingPointOverride=on  logOutputs=off  logFile=C:\Users\ASUS\Desktop\sift_fpga_final\Octave_2\tb_test\test_octave2_dog%5Fspace_Parallel+Adder+Subtractor.fixedpointlog
  Parallel Adder Subtractor1 : allblocks_alteradspbuilder2/Parallel Adder Subtractor  number_of_inputs=2  direction=+-  use_pipeline=on  pipeline_display=1  phase_selection=1  use_ena=on  use_aclr=off  allowFloatingPointOverride=on  logOutputs=off  logFile=C:\Users\ASUS\Desktop\sift_fpga_final\Octave_2\tb_test\test_octave2_dog%5Fspace_Parallel+Adder+Subtractor1.fixedpointlog
  Parallel Adder Subtractor2 : allblocks_alteradspbuilder2/Parallel Adder Subtractor  number_of_inputs=2  direction=+-  use_pipeline=on  pipeline_display=1  phase_selection=1  use_ena=on  use_aclr=off  allowFloatingPointOverride=on  logOutputs=off  logFile=C:\Users\ASUS\Desktop\sift_fpga_final\Octave_2\tb_test\test_octave2_dog%5Fspace_Parallel+Adder+Subtractor2.fixedpointlog
  dog3_out : Outport
  dog2_out : Outport  Port=2
  dog1_out : Outport  Port=3
  wires:
  [pixel_scale2] -> Parallel Adder Subtractor1/1
  Parallel Adder Subtractor1/1 -> dog1_out/1
  [pixel_scale3] -> Parallel Adder Subtractor/1
  [valid_in] -> Parallel Adder Subtractor2/3
  [pixel_scale2] -> Parallel Adder Subtractor/2
  [pixel_scale3] -> Parallel Adder Subtractor2/2
  Parallel Adder Subtractor/1 -> dog2_out/1
  [valid_in] -> Parallel Adder Subtractor1/3
  Parallel Adder Subtractor2/1 -> dog3_out/1
  [pixel_scale1] -> Parallel Adder Subtractor1/2
  [valid_in] -> Parallel Adder Subtractor/3
  [pixel_scale4] -> Parallel Adder Subtractor2/1
  scale4_in/1 -> [pixel_scale4]
  scale3_in/1 -> [pixel_scale3]
  scale2_in/1 -> [pixel_scale2]
  scale1_in/1 -> [pixel_scale1]
  valid_in/1 -> [valid_in]
